simulink model "DYC_DLCtight_Fuzzy_and_NN_prediction"  (Simulink 8.9)
settings: Solver=VariableStepAuto  StartTime=0  StopTime=8  FixedStep=0.001  RelTol=1e-3  AbsTol=1e-6
libraries: neural x138, fuzblock x6, dspfdesign x6, Solver_SF x1, simulink x1
(part 1 of 4)
settings Model: Creator=ywata  LastModifiedBy=Huang Guoming  ExtModeTrigMode=oneshot  ExtModeArmWhenConnect=off
settings Model: LogicAnalyzerGraphicalSettings=|
  | {
  |   "cursors" : {
  |     "activeCursor" : 1,
  |     "lockedCursors" : [
  | 
  |     ],
  |     "startingCursor" : 0,
  |     "times" : [
  |       1.76,
  |       0.487,
  |       1.4983333333333333
  |     ]
  |   },
  |   "global" : {
  |   },
  |   "panels" : [
  |     {
  |       "height" : 100,
  |       "startingTrace" : 0,
  |       "traces" : [
  | 
  |       ],
  |       "yOffset" : 0
  |     }
  |   ],
  |   "timeAxis" : {
  |     "pixelsPerSecond" : 300
  |   }
  | }
settings DataIOCC: LimitDataPoints=off  SignalLoggingName=sigsOut
settings OptimizationCC: BooleanDataType=off
settings DebuggingCC: SaveWithParameterizedLinksMsg=none  SignalResolutionControl=TryResolveAllWithWarning  MultiTaskDSMMsg=warning  MultiTaskCondExecSysMsg=none
settings HardwareCC: TargetBitPerPointer=64  TargetBitPerSizeT=64  TargetBitPerPtrDiffT=64  TargetLongLongMode=on  TargetIntDivRoundTo=Zero  TargetEndianess=LittleEndian  TargetWordSize=64  TargetHWDeviceType=MATLAB Host  ProdEqTarget=off
settings RTWCC: TemplateMakefile=grt_vc.tmf
settings GRTTargetCC: GeneratePreprocessorConditionals=Use local settings

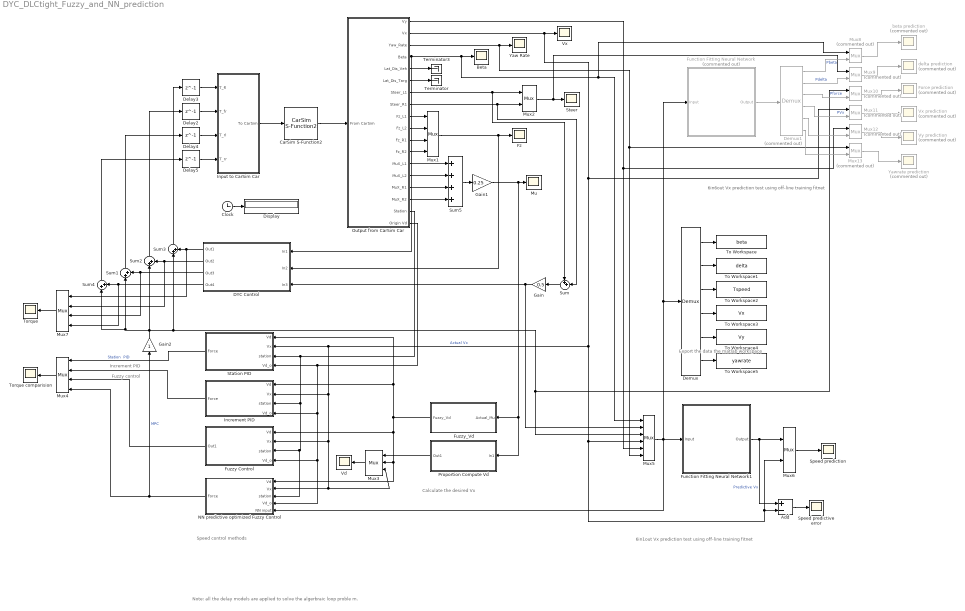
== system DYC_DLCtight_Fuzzy_and_NN_prediction ==
  note: Fuzzy control
  note: Increment PID
  note: Calculate the desired Vx
  note: Speed control methods
  note: Export the data the matlab workspace
  note: Note: all the delay models are applied to solve the algerbraic loop proble m.
  note: 6in1out Vx prediction test using off-line training fitnet
  note: 6in6out Vx prediction test using off-line training fitnet
  " Force prediction" : Scope  Commented=on
  " Fuzzy Control" : Subsystem
      mask Display: image('fuzzy.jpg');
  " Vx prediction" : Scope  Commented=on
  " Vy prediction" : Scope  Commented=on
  " Yawrate prediction" : Scope  Commented=on
  " beta prediction" : Scope  Commented=on
  " delta prediction" : Scope  Commented=on
  Add : Sum  Inputs=+-
  Beta : Scope
  CarSim S-Function2 : Solver_SF/CarSim S-Function2  Priority=1  VehicleCode=i_i  SIMFILE=simfile.sim
      settings: AttributesFormatString=Vehicle Code: %<VehicleCode>
  Clock : Clock
  DYC Control : Subsystem
  Delay{2..5} (4 alike) : Delay  DelayLength=1  InitialCondition=0  SampleTime=0.001
  Demux : Demux  Outputs=6
  Demux1 : Demux  Commented=on  Outputs=6
  Display : Display
      settings: Format=bank  Decimation=100
  Function Fitting Neural Network : Subsystem  Commented=on
      mask help: Function Fitting Neural Network
      mask Display: e = 0.06;c1 = [120 150 230]/255;c2 = ([120 150 230]+0)/383;c3 = ([120 150 230]+128)/383;patch([0 1 1 0],[0 0 1 1],c1);patch([0 1 1 1-e 1-e 0+e],[0 0 1 1-e 0+e 0+e],c2);patch([0 0 1 1-e 0+e 0+e],[0 1 1 1-e 1-e 0+e],c3);plot([0 1 1 0 0],[0 0 1 1 0]);fprintf('NNET');port_label('input',1,' Input');port_label('output',1,'Output ');
  Function Fitting Neural Network1 : Subsystem
      mask help: Function Fitting Neural Network
      mask Display: e = 0.06;c1 = [120 150 230]/255;c2 = ([120 150 230]+0)/383;c3 = ([120 150 230]+128)/383;patch([0 1 1 0],[0 0 1 1],c1);patch([0 1 1 1-e 1-e 0+e],[0 0 1 1-e 0+e 0+e],c2);patch([0 0 1 1-e 0+e 0+e],[0 1 1 1-e 1-e 0+e],c3);plot([0 1 1 0 0],[0 0 1 1 0]);fprintf('NNET');port_label('input',1,' Input');port_label('output',1,'Output ');
  Fuzzy_Vd : MATLAB Function  TreatAsAtomicUnit=on
  Fz : Scope
  Gain : Gain  Gain=0.5
  Gain1 : Gain  Gain=0.25
  Gain2 : Gain
  "Increment PID " : Subsystem
  Input to CarSim Car : Subsystem
  Mu : Scope
  Mux1 : Mux
  Mux{8..13} (6 alike) : Mux  Commented=on  Inputs=2
  Mux2 : Mux  Inputs=2
  Mux3 : Mux  Inputs=3
  Mux4 : Mux
  Mux5 : Mux  Inputs=6
  Mux6 : Mux  Inputs=2
  Mux7 : Mux
  NN predictive optimized Fuzzy Control : Subsystem
  Output from CarSim Car : Subsystem
  Proportion Compute Vd : Subsystem
  Speed prediction : Scope
  Speed predictive error : Scope
  Station PID : Subsystem
  Steer : Scope
  Sum : Sum  Inputs=++|
  Sum{1..4} (4 alike) : Sum  Inputs=|++
  Sum5 : Sum  Inputs=++++
  Terminator : Terminator
  Terminator3 : Terminator
  To Workspace : ToWorkspace  VariableName=beta  SampleTime=-1
      settings: Save2DSignal=2-D array (concatenate along first dimension)
  To Workspace1 : ToWorkspace  VariableName=delta  SampleTime=-1
      settings: Save2DSignal=2-D array (concatenate along first dimension)
  To Workspace2 : ToWorkspace  VariableName=Tspeed  SampleTime=-1
      settings: Save2DSignal=2-D array (concatenate along first dimension)
  To Workspace3 : ToWorkspace  VariableName=Vx  SampleTime=-1
      settings: Save2DSignal=2-D array (concatenate along first dimension)
  To Workspace4 : ToWorkspace  VariableName=Vy  SampleTime=-1
      settings: Save2DSignal=2-D array (concatenate along first dimension)
  To Workspace5 : ToWorkspace  VariableName=yawrate  SampleTime=-1
      settings: Save2DSignal=2-D array (concatenate along first dimension)
  Torque : Scope
  Torque comparision : Scope
  Vd : Scope
  Vx : Scope
  Yaw Rate : Scope
  wires:
  Clock/1 -> Display/1
  Mux2/1 -> Mux9/1, Steer/1
  Mux7/1 -> Torque/1
  Output from CarSim Car/3(Yaw_Rate) -> Mux5/6, Mux13/1, Yaw Rate/1
  Output from CarSim Car/6(Lat_Dis_Targ) -> Terminator/1
  Output from CarSim Car/5(Lat_Dis_Veh) -> Terminator3/1
  Output from CarSim Car/1(Vy) -> Mux5/5, Mux12/1
  Output from CarSim Car/4(Beta) -> Mux8/1, Mux5/1, Beta/1, DYC Control/1(In1)
  Output from CarSim Car/7(Steer_L1) -> Sum/1, Mux2/1
  Output from CarSim Car/8(Steer_R1) -> Sum/2, Mux2/2
  Output from CarSim Car/2(Vx) -> Mux11/1, Mux3/3, NN predictive optimized Fuzzy Control/2(Vx), " Fuzzy Control"/2(Vx), "Increment PID "/2(Vx), Station PID/2(Vx), Mux5/4, Mux6/2, Add/2, Vx/1  "Actual Vx"
  Sum/1 -> Gain/1
  Sum3/1 -> Delay3/1
  Sum2/1 -> Delay2/1
  Sum4/1 -> Delay5/1
  Output from CarSim Car/13(MuX_L1) -> Sum5/1
  Output from CarSim Car/14(MuX_L2) -> Sum5/2
  Output from CarSim Car/15(MuX_R1) -> Sum5/3
  Output from CarSim Car/16(MuX_R2) -> Sum5/4
  Sum5/1 -> Gain1/1
  Gain1/1 -> Mu/1, Fuzzy_Vd/1(Actual_Mu), Proportion Compute Vd/1(In1)
  CarSim S-Function2/1 -> Output from CarSim Car/1(From CarSim)
  Input to CarSim Car/1(To CarSim) -> CarSim S-Function2/1
  Output from CarSim Car/9(Fz_L1) -> Mux1/1
  Output from CarSim Car/10(Fz_L2) -> Mux1/2
  Output from CarSim Car/11(Fz_R1) -> Mux1/3
  Output from CarSim Car/12(Fz_R2) -> Mux1/4
  Mux1/1 -> DYC Control/2(In2), Fz/1
  Mux3/1 -> Vd/1
  Proportion Compute Vd/1(Out1) -> Mux3/1
  Mux4/1 -> Torque comparision/1
  Delay3/1 -> Input to CarSim Car/1(T_fl)
  Delay2/1 -> Input to CarSim Car/2(T_fr)
  Delay4/1 -> Input to CarSim Car/3(T_rl)
  Delay5/1 -> Input to CarSim Car/4(T_rr)
  DYC Control/2(Out2) -> Sum2/2, Mux7/2
  DYC Control/4(Out4) -> Sum4/2, Mux7/4
  DYC Control/1(Out1) -> Sum3/2, Mux7/1
  DYC Control/3(Out3) -> Sum1/2, Mux7/3
  Gain/1 -> Mux5/2, DYC Control/3(In3)
  Station PID/1(Force) -> Mux4/1  "Station  PID"
  Sum1/1 -> Delay4/1
  Function Fitting Neural Network1/1(Output) -> Add/1, Mux6/1  "Predictive Vx"
  Mux6/1 -> Speed prediction/1
  " Fuzzy Control"/1(Out1) -> Mux4/3
  Demux/5 -> To Workspace4/1
  Demux/4 -> To Workspace3/1
  Demux/3 -> To Workspace2/1
  Demux/2 -> To Workspace1/1
  Demux/1 -> To Workspace/1
  Demux/6 -> To Workspace5/1
  Mux5/1 -> Function Fitting Neural Network/1(Input), Demux/1, NN predictive optimized Fuzzy Control/5(NN input), Function Fitting Neural Network1/1(Input)
  Gain2/1 -> Sum4/1, Sum1/1, Sum2/1, Mux10/1, Mux5/3, Sum3/1
  "Increment PID "/1(Force) -> Mux4/2
  Add/1 -> Speed predictive error/1
  Fuzzy_Vd/1(Fuzzy_Vd) -> Station PID/1(Vd), "Increment PID "/1(Vd), NN predictive optimized Fuzzy Control/1(Vd), Mux3/2, " Fuzzy Control"/1(Vd)
  Output from CarSim Car/18(Origin Vd) -> NN predictive optimized Fuzzy Control/4(Vd_o), " Fuzzy Control"/4(Vd_o), "Increment PID "/4(Vd_o), Station PID/4(Vd_o)
  Output from CarSim Car/17(Station) -> NN predictive optimized Fuzzy Control/3(station), " Fuzzy Control"/3(station), "Increment PID "/3(station), Station PID/3(station)
  NN predictive optimized Fuzzy Control/1(Force) -> Gain2/1, Mux4/4  "MPC"
  Function Fitting Neural Network/1(Output) -> Demux1/1
  Mux8/1 -> " beta prediction"/1
  Demux1/1 -> Mux8/2  "Pbeta"
  Demux1/2 -> Mux9/2  "Pdelta"
  Mux9/1 -> " delta prediction"/1
  Demux1/3 -> Mux10/2  "Pforce"
  Mux10/1 -> " Force prediction"/1
  Demux1/4 -> Mux11/2  "PVx"
  Mux11/1 -> " Vx prediction"/1
  Demux1/5 -> Mux12/2
  Mux12/1 -> " Vy prediction"/1
  Demux1/6 -> Mux13/2
  Mux13/1 -> " Yawrate prediction"/1

== system DYC_DLCtight_Fuzzy_and_NN_prediction/ Fuzzy Control ==
  Vd : Inport
  Vx : Inport  Port=2
  station : Inport  Port=3
  Vd_o : Inport  Port=4
  Fuzzy control : Subsystem
  Select Vd : MATLAB Function  TreatAsAtomicUnit=on
  Out1 : Outport
  wires:
  Fuzzy control/1(Out1) -> Out1/1
  Select Vd/1(Ve) -> Fuzzy control/1(In1)
  Vd/1 -> Select Vd/1(Vd)
  Vx/1 -> Select Vd/2(Vx)
  station/1 -> Select Vd/3(station)
  Vd_o/1 -> Select Vd/4(Vd_o)

== system DYC_DLCtight_Fuzzy_and_NN_prediction/DYC Control ==
  In1 : Inport
  In2 : Inport  Port=2
  In3 : Inport  Port=3
  DYC  control method : MATLAB Function  TreatAsAtomicUnit=on
  Demux : Demux
  Out1 : Outport
  Out2 : Outport  Port=2
  Out3 : Outport  Port=3
  Out4 : Outport  Port=4
  wires:
  In3/1 -> DYC  control method/1(delta)
  DYC  control method/1(T1) -> Out1/1
  Demux/2 -> DYC  control method/4(Fz_fr)
  DYC  control method/4(T4) -> Out4/1
  Demux/1 -> DYC  control method/3(Fz_fl)
  Demux/4 -> DYC  control method/6(Fz_rr)
  DYC  control method/3(T3) -> Out3/1
  DYC  control method/2(T2) -> Out2/1
  Demux/3 -> DYC  control method/5(Fz_rl)
  In2/1 -> Demux/1
  In1/1 -> DYC  control method/2(beta)

== system DYC_DLCtight_Fuzzy_and_NN_prediction/Function Fitting Neural Network ==
  Input : Inport  PortDimensions=6
      mask Display: e = 0.06;c1 = [120 230 180]/255;c2 = ([120 230 180]+0)/(256+128);c3 = ([120 230 180]+128)/(256+128);patch([0 1 1 0],[0 0 1 1],c1);patch([0 1 1 1-e 1-e 0+e],[0 0 1 1-e 0+e 0+e],c2);patch([0 0 1 1-e 0+e 0+e],[0 1 1 1-e 1-e 0+e],c3);plot([0 1 1 0 0],[0 0 1 1 0]);
  Layer 1 : Subsystem
      mask Display: e = 0.06;c1 = [120 150 230]/255;c2 = ([120 150 230]+0)/383;c3 = ([120 150 230]+128)/383;patch([0 1 1 0],[0 0 1 1],c1);patch([0 1 1 1-e 1-e 0+e],[0 0 1 1-e 0+e 0+e],c2);patch([0 0 1 1-e 0+e 0+e],[0 1 1 1-e 1-e 0+e],c3);plot([0 1 1 0 0],[0 0 1 1 0]);
  Layer 2 : Subsystem
      mask Display: e = 0.06;c1 = [120 150 230]/255;c2 = ([120 150 230]+0)/383;c3 = ([120 150 230]+128)/383;patch([0 1 1 0],[0 0 1 1],c1);patch([0 1 1 1-e 1-e 0+e],[0 0 1 1-e 0+e 0+e],c2);patch([0 0 1 1-e 0+e 0+e],[0 1 1 1-e 1-e 0+e],c3);plot([0 1 1 0 0],[0 0 1 1 0]);
  Process Input 1 : Subsystem
      mask Display: e = 0.06;c1 = [120 150 230]/255;c2 = ([120 150 230]+0)/383;c3 = ([120 150 230]+128)/383;patch([0 1 1 0],[0 0 1 1],c1);patch([0 1 1 1-e 1-e 0+e],[0 0 1 1-e 0+e 0+e],c2);patch([0 0 1 1-e 0+e 0+e],[0 1 1 1-e 1-e 0+e],c3);plot([0 1 1 0 0],[0 0 1 1 0]);
  Process Output 1 : Subsystem
      mask Display: e = 0.06;c1 = [120 150 230]/255;c2 = ([120 150 230]+0)/383;c3 = ([120 150 230]+128)/383;patch([0 1 1 0],[0 0 1 1],c1);patch([0 1 1 1-e 1-e 0+e],[0 0 1 1-e 0+e 0+e],c2);patch([0 0 1 1-e 0+e 0+e],[0 1 1 1-e 1-e 0+e],c3);plot([0 1 1 0 0],[0 0 1 1 0]);
  Output : Outport  InitialOutput=[0;0;0;0;0;0]
      mask Display: e = 0.06;c1 = [120 230 180]/255;c2 = ([120 230 180]+0)/(256+128);c3 = ([120 230 180]+128)/(256+128);patch([0 1 1 0],[0 0 1 1],c1);patch([0 1 1 1-e 1-e 0+e],[0 0 1 1-e 0+e 0+e],c2);patch([0 0 1 1-e 0+e 0+e],[0 1 1 1-e 1-e 0+e],c3);plot([0 1 1 0 0],[0 0 1 1 0]);
  wires:
  Input/1 -> Process Input 1/1(x)
  Process Output 1/1(y) -> Output/1
  Process Input 1/1(p) -> Layer 1/1("p{1}")
  Layer 1/1("a{1}") -> [feedback1]
  [feedback1] -> Layer 2/1("a{1} ")
  Layer 2/1("a{2}") -> Process Output 1/1(a)

== system DYC_DLCtight_Fuzzy_and_NN_prediction/Function Fitting Neural Network1 ==
  Input : Inport  PortDimensions=6
      mask Display: e = 0.06;c1 = [120 230 180]/255;c2 = ([120 230 180]+0)/(256+128);c3 = ([120 230 180]+128)/(256+128);patch([0 1 1 0],[0 0 1 1],c1);patch([0 1 1 1-e 1-e 0+e],[0 0 1 1-e 0+e 0+e],c2);patch([0 0 1 1-e 0+e 0+e],[0 1 1 1-e 1-e 0+e],c3);plot([0 1 1 0 0],[0 0 1 1 0]);
  Layer 1 : Subsystem
      mask Display: e = 0.06;c1 = [120 150 230]/255;c2 = ([120 150 230]+0)/383;c3 = ([120 150 230]+128)/383;patch([0 1 1 0],[0 0 1 1],c1);patch([0 1 1 1-e 1-e 0+e],[0 0 1 1-e 0+e 0+e],c2);patch([0 0 1 1-e 0+e 0+e],[0 1 1 1-e 1-e 0+e],c3);plot([0 1 1 0 0],[0 0 1 1 0]);
  Layer 2 : Subsystem
      mask Display: e = 0.06;c1 = [120 150 230]/255;c2 = ([120 150 230]+0)/383;c3 = ([120 150 230]+128)/383;patch([0 1 1 0],[0 0 1 1],c1);patch([0 1 1 1-e 1-e 0+e],[0 0 1 1-e 0+e 0+e],c2);patch([0 0 1 1-e 0+e 0+e],[0 1 1 1-e 1-e 0+e],c3);plot([0 1 1 0 0],[0 0 1 1 0]);
  Process Input 1 : Subsystem
      mask Display: e = 0.06;c1 = [120 150 230]/255;c2 = ([120 150 230]+0)/383;c3 = ([120 150 230]+128)/383;patch([0 1 1 0],[0 0 1 1],c1);patch([0 1 1 1-e 1-e 0+e],[0 0 1 1-e 0+e 0+e],c2);patch([0 0 1 1-e 0+e 0+e],[0 1 1 1-e 1-e 0+e],c3);plot([0 1 1 0 0],[0 0 1 1 0]);
  Process Output 1 : Subsystem
      mask Display: e = 0.06;c1 = [120 150 230]/255;c2 = ([120 150 230]+0)/383;c3 = ([120 150 230]+128)/383;patch([0 1 1 0],[0 0 1 1],c1);patch([0 1 1 1-e 1-e 0+e],[0 0 1 1-e 0+e 0+e],c2);patch([0 0 1 1-e 0+e 0+e],[0 1 1 1-e 1-e 0+e],c3);plot([0 1 1 0 0],[0 0 1 1 0]);
  Output : Outport  InitialOutput=0
      mask Display: e = 0.06;c1 = [120 230 180]/255;c2 = ([120 230 180]+0)/(256+128);c3 = ([120 230 180]+128)/(256+128);patch([0 1 1 0],[0 0 1 1],c1);patch([0 1 1 1-e 1-e 0+e],[0 0 1 1-e 0+e 0+e],c2);patch([0 0 1 1-e 0+e 0+e],[0 1 1 1-e 1-e 0+e],c3);plot([0 1 1 0 0],[0 0 1 1 0]);
  wires:
  Input/1 -> Process Input 1/1(x)
  Process Output 1/1(y) -> Output/1
  Process Input 1/1(p) -> Layer 1/1("p{1}")
  Layer 1/1("a{1}") -> [feedback1]
  [feedback1] -> Layer 2/1("a{1} ")
  Layer 2/1("a{2}") -> Process Output 1/1(a)

== system DYC_DLCtight_Fuzzy_and_NN_prediction/Increment PID  ==
  Vd : Inport
  Vx : Inport  Port=2
  station : Inport  Port=3
  Vd_o : Inport  Port=4
  "Increment PID " : Subsystem
  Select Vd : MATLAB Function  TreatAsAtomicUnit=on
  Force : Outport
  wires:
  "Increment PID "/1(Out1) -> Force/1
  Select Vd/1(Ve) -> "Increment PID "/1(In1)
  Vd/1 -> Select Vd/1(Vd)
  Vx/1 -> Select Vd/2(Vx)
  station/1 -> Select Vd/3(station)
  Vd_o/1 -> Select Vd/4(Vd_o)

== system DYC_DLCtight_Fuzzy_and_NN_prediction/Input to CarSim Car ==
  T_fl : Inport
  T_fr : Inport  Port=2
  T_rl : Inport  Port=3
  T_rr : Inport  Port=4
  Mux : Mux
  To CarSim : Outport
  wires:
  T_rr/1 -> Mux/4
  T_rl/1 -> Mux/3
  T_fr/1 -> Mux/2
  T_fl/1 -> Mux/1
  Mux/1 -> To CarSim/1

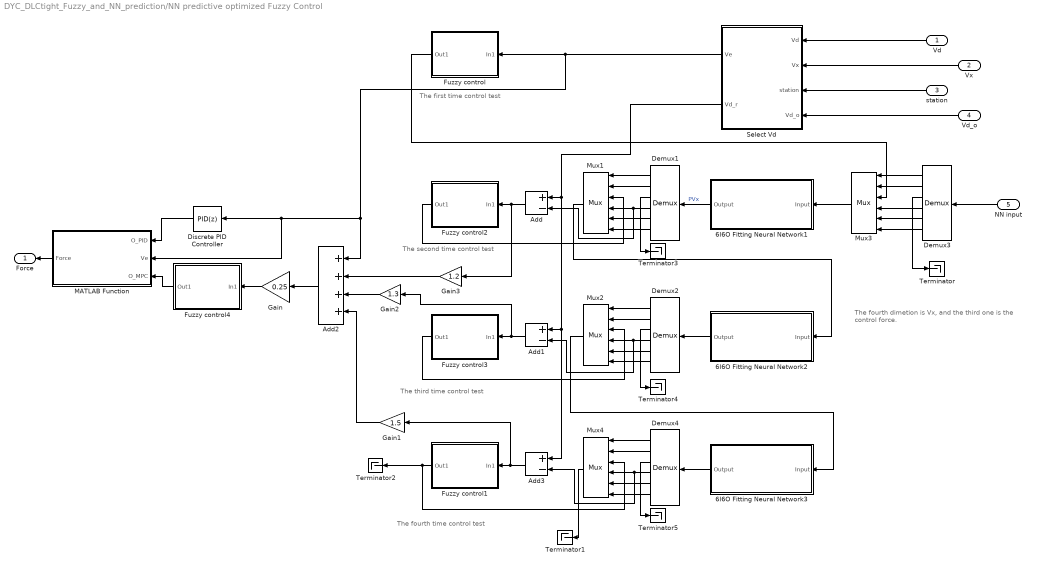
== system DYC_DLCtight_Fuzzy_and_NN_prediction/NN predictive optimized Fuzzy Control ==
  note: The first time control test
  note: The fourth dimetion is Vx,
      | and the third one is the control force.
  note: The second time control test
  note: The third time control test
  note: The fourth time control test
  Vd : Inport
  Vx : Inport  Port=2
  station : Inport  Port=3
  Vd_o : Inport  Port=4
  NN input : Inport  Port=5
  6I6O Fitting Neural Network1 : Subsystem
      mask help: Function Fitting Neural Network
      mask Display: e = 0.06;c1 = [120 150 230]/255;c2 = ([120 150 230]+0)/383;c3 = ([120 150 230]+128)/383;patch([0 1 1 0],[0 0 1 1],c1);patch([0 1 1 1-e 1-e 0+e],[0 0 1 1-e 0+e 0+e],c2);patch([0 0 1 1-e 0+e 0+e],[0 1 1 1-e 1-e 0+e],c3);plot([0 1 1 0 0],[0 0 1 1 0]);fprintf('NNET');port_label('input',1,' Input');port_label('output',1,'Output ');
  6I6O Fitting Neural Network2 : Subsystem
      mask help: Function Fitting Neural Network
      mask Display: e = 0.06;c1 = [120 150 230]/255;c2 = ([120 150 230]+0)/383;c3 = ([120 150 230]+128)/383;patch([0 1 1 0],[0 0 1 1],c1);patch([0 1 1 1-e 1-e 0+e],[0 0 1 1-e 0+e 0+e],c2);patch([0 0 1 1-e 0+e 0+e],[0 1 1 1-e 1-e 0+e],c3);plot([0 1 1 0 0],[0 0 1 1 0]);fprintf('NNET');port_label('input',1,' Input');port_label('output',1,'Output ');
  6I6O Fitting Neural Network3 : Subsystem
      mask help: Function Fitting Neural Network
      mask Display: e = 0.06;c1 = [120 150 230]/255;c2 = ([120 150 230]+0)/383;c3 = ([120 150 230]+128)/383;patch([0 1 1 0],[0 0 1 1],c1);patch([0 1 1 1-e 1-e 0+e],[0 0 1 1-e 0+e 0+e],c2);patch([0 0 1 1-e 0+e 0+e],[0 1 1 1-e 1-e 0+e],c3);plot([0 1 1 0 0],[0 0 1 1 0]);fprintf('NNET');port_label('input',1,' Input');port_label('output',1,'Output ');
  Add : Sum  Inputs=+-
  Add1 : Sum  Inputs=+-
  Add2 : Sum  Inputs=++++
  Add3 : Sum  Inputs=+-
  Demux{1..4} (4 alike) : Demux  Outputs=6
  Discrete PID Controller : simulink/Continuous/PID Controller  Controller=PID  TimeDomain=Discrete-time  SampleTime=-1  IntegratorMethod=Forward Euler  FilterMethod=Forward Euler  Form=Parallel  UseFilter=on  ControllerParametersSource=internal  P=500  I=0  D=200  N=100  InitialConditionSource=internal  InitialConditionForIntegrator=0  InitialConditionForFilter=0  ExternalReset=none  LimitOutput=off  UpperSaturationLimit=inf  LowerSaturationLimit=-inf  LinearizeAsGain=off  AntiWindupMode=none  Kb=1  TrackingMode=off  Kt=1  PParamMin=[]  PParamMax=[]  IParamMin=[]  IParamMax=[]  DParamMin=[]  DParamMax=[]  NParamMin=[]  NParamMax=[]  KbParamMin=[]  KbParamMax=[]  KtParamMin=[]  KtParamMax=[]  POutMin=[]  POutMax=[]  IOutMin=[]  IOutMax=[]  DOutMin=[]  DOutMax=[]  NOutMin=[]  NOutMax=[]  KbOutMin=[]  KbOutMax=[]  KtOutMin=[]  KtOutMax=[]  IntegratorOutMin=[]  IntegratorOutMax=[]  FilterOutMin=[]  FilterOutMax=[]  SumOutMin=[]  SumOutMax=[]  SumI1OutMin=[]  SumI1OutMax=[]  SumI2OutMin=[]  SumI2OutMax=[]  SumI3OutMin=[]  SumI3OutMax=[]  SumDOutMin=[]  SumDOutMax=[]  SaturationOutMin=[]  SaturationOutMax=[]  IntegratorContinuousStateAttributes=''  IntegratorStateMustResolveToSignalObject=off  IntegratorRTWStateStorageClass=Auto  FilterContinuousStateAttributes=''  FilterStateMustResolveToSignalObject=off  FilterRTWStateStorageClass=Auto  DifferentiatorICPrevScaledInput=0  DifferentiatorOutMin=[]  DifferentiatorOutMax=[]  InitialConditionSetting=State (most efficient)
  Fuzzy control : Subsystem
  Fuzzy control1 : Subsystem
  Fuzzy control2 : Subsystem
  Fuzzy control3 : Subsystem
  Fuzzy control4 : Subsystem
  Gain : Gain  Gain=0.25
  Gain1 : Gain  Gain=1.5
  Gain2 : Gain  Gain=1.3
  Gain3 : Gain  Gain=1.2
  MATLAB Function : MATLAB Function  TreatAsAtomicUnit=on
  Mux{1..4} (4 alike) : Mux  Inputs=6
  Select Vd : MATLAB Function  TreatAsAtomicUnit=on
  Terminator{,1..5} (6 alike) : Terminator
  Force : Outport
  wires:
  Vd_o/1 -> Select Vd/4(Vd_o)
  station/1 -> Select Vd/3(station)
  Vx/1 -> Select Vd/2(Vx)
  Vd/1 -> Select Vd/1(Vd)
  6I6O Fitting Neural Network1/1(Output) -> Demux1/1  "PVx"
  Mux1/1 -> 6I6O Fitting Neural Network2/1(Input)
  Demux1/6 -> Mux1/6
  Demux1/5 -> Mux1/5
  Demux1/2 -> Mux1/2
  Demux1/1 -> Mux1/1
  Select Vd/1(Ve) -> MATLAB Function/2(Ve), Discrete PID Controller/1, Add2/1, Fuzzy control/1(In1)
  Demux2/1 -> Mux2/1
  Demux2/2 -> Mux2/2
  Demux2/5 -> Mux2/5
  Demux2/6 -> Mux2/6
  6I6O Fitting Neural Network2/1(Output) -> Demux2/1
  NN input/1 -> Demux3/1
  Mux3/1 -> 6I6O Fitting Neural Network1/1(Input)
  Demux3/5 -> Mux3/5
  Demux3/6 -> Mux3/6
  Demux3/2 -> Mux3/2
  Demux3/1 -> Mux3/1
  Add/1 -> Gain3/1, Fuzzy control2/1(In1)
  Add1/1 -> Gain2/1, Fuzzy control3/1(In1)
  6I6O Fitting Neural Network3/1(Output) -> Demux4/1
  Demux4/6 -> Mux4/6
  Demux4/5 -> Mux4/5
  Demux4/2 -> Mux4/2
  Demux4/1 -> Mux4/1
  Mux2/1 -> 6I6O Fitting Neural Network3/1(Input)
  Select Vd/2(Vd_r) -> Add1/1, Add3/1, Add/1
  Add3/1 -> Gain1/1, Fuzzy control1/1(In1)
  Mux4/1 -> Terminator1/1
  Add2/1 -> Gain/1
  Gain/1 -> Fuzzy control4/1(In1)
  Demux2/4 -> Add1/2, Mux2/4
  Fuzzy control3/1(Out1) -> Mux2/3
  Demux4/4 -> Add3/2, Mux4/4
  Fuzzy control/1(Out1) -> Mux3/3
  Demux3/4 -> Mux3/4
  Demux3/3 -> Terminator/1
  Fuzzy control2/1(Out1) -> Mux1/3
  Fuzzy control1/1(Out1) -> Mux4/3, Terminator2/1
  Demux1/4 -> Mux1/4, Add/2
  Demux1/3 -> Terminator3/1
  Demux2/3 -> Terminator4/1
  Demux4/3 -> Terminator5/1
  Gain1/1 -> Add2/4
  Gain2/1 -> Add2/3
  Gain3/1 -> Add2/2
  Fuzzy control4/1(Out1) -> MATLAB Function/3(O_MPC)
  MATLAB Function/1(Force) -> Force/1
  Discrete PID Controller/1 -> MATLAB Function/1(O_PID)

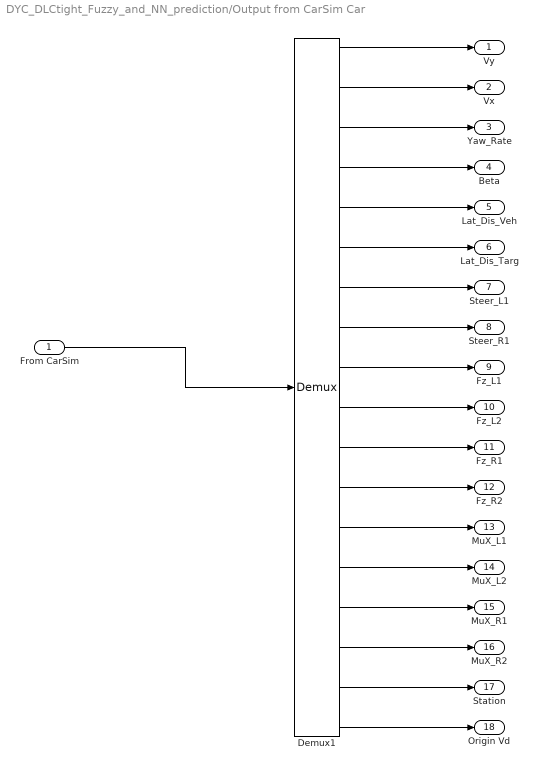
== system DYC_DLCtight_Fuzzy_and_NN_prediction/Output from CarSim Car ==
  From CarSim : Inport
  Demux1 : Demux  Outputs=18
  Vy : Outport
  Vx : Outport  Port=2
  Yaw_Rate : Outport  Port=3
  Beta : Outport  Port=4
  Lat_Dis_Veh : Outport  Port=5
  Lat_Dis_Targ : Outport  Port=6
  Steer_L1 : Outport  Port=7
  Steer_R1 : Outport  Port=8
  Fz_L1 : Outport  Port=9
  Fz_L2 : Outport  Port=10
  Fz_R1 : Outport  Port=11
  Fz_R2 : Outport  Port=12
  MuX_L1 : Outport  Port=13
  MuX_L2 : Outport  Port=14
  MuX_R1 : Outport  Port=15
  MuX_R2 : Outport  Port=16
  Station : Outport  Port=17
  Origin Vd : Outport  Port=18
  wires:
  From CarSim/1 -> Demux1/1
  Demux1/2 -> Vx/1
  Demux1/3 -> Yaw_Rate/1
  Demux1/1 -> Vy/1
  Demux1/8 -> Steer_R1/1
  Demux1/4 -> Beta/1
  Demux1/5 -> Lat_Dis_Veh/1
  Demux1/6 -> Lat_Dis_Targ/1
  Demux1/7 -> Steer_L1/1
  Demux1/9 -> Fz_L1/1
  Demux1/10 -> Fz_L2/1
  Demux1/11 -> Fz_R1/1
  Demux1/12 -> Fz_R2/1
  Demux1/13 -> MuX_L1/1
  Demux1/14 -> MuX_L2/1
  Demux1/15 -> MuX_R1/1
  Demux1/16 -> MuX_R2/1
  Demux1/17 -> Station/1
  Demux1/18 -> Origin Vd/1

== system DYC_DLCtight_Fuzzy_and_NN_prediction/Proportion Compute Vd ==
  In1 : Inport
  Constant : Constant  Value=0.45
  Constant1 : Constant  Value=30
  Gain : Gain  Gain=50
  Sum : Sum  Inputs=|+-
  Sum1 : Sum
  Out1 : Outport
  wires:
  In1/1 -> Sum/1
  Constant/1 -> Sum/2
  Sum/1 -> Gain/1
  Gain/1 -> Sum1/1
  Sum1/1 -> Out1/1
  Constant1/1 -> Sum1/2

== system DYC_DLCtight_Fuzzy_and_NN_prediction/Station PID ==
  Vd : Inport
  Vx : Inport  Port=2
  station : Inport  Port=3
  Vd_o : Inport  Port=4
  " PID speed control method" : MATLAB Function  TreatAsAtomicUnit=on
  Force : Outport
  wires:
  " PID speed control method"/1(BrakeTorque) -> Force/1
  Vd/1 -> " PID speed control method"/1(Vd)
  Vx/1 -> " PID speed control method"/2(Vx)
  Vd_o/1 -> " PID speed control method"/4(Vd_o)
  station/1 -> " PID speed control method"/3(station)

== system DYC_DLCtight_Fuzzy_and_NN_prediction/ Fuzzy Control/Fuzzy control ==
  In1 : Inport
  Fuzzy Logic  Controller : fuzblock/Fuzzy Logic  Controller  fis='FuzzyInferenceSystem.fis'
  Gain3 : Gain  Gain=120
  Signal pre-process : Subsystem
  Out1 : Outport
  wires:
  Gain3/1 -> Out1/1
  Signal pre-process/1(Out1) -> Fuzzy Logic  Controller/1
  In1/1 -> Signal pre-process/1(In1)
  Fuzzy Logic  Controller/1 -> Gain3/1

== system DYC_DLCtight_Fuzzy_and_NN_prediction/Function Fitting Neural Network/Layer 1 ==
  "p{1}" : Inport  PortDimensions=6
      mask Display: e = 0.06;c1 = [120 230 180]/255;c2 = ([120 230 180]+0)/(256+128);c3 = ([120 230 180]+128)/(256+128);patch([0 1 1 0],[0 0 1 1],c1);patch([0 1 1 1-e 1-e 0+e],[0 0 1 1-e 0+e 0+e],c2);patch([0 0 1 1-e 0+e 0+e],[0 1 1 1-e 1-e 0+e],c3);plot([0 1 1 0 0],[0 0 1 1 0]);
  Delays 1 : Subsystem
      mask Display: e = 0.06;c1 = [120 150 230]/255;c2 = ([120 150 230]+0)/383;c3 = ([120 150 230]+128)/383;patch([0 1 1 0],[0 0 1 1],c1);patch([0 1 1 1-e 1-e 0+e],[0 0 1 1-e 0+e 0+e],c2);patch([0 0 1 1-e 0+e 0+e],[0 1 1 1-e 1-e 0+e],c3);plot([0 1 1 0 0],[0 0 1 1 0]);disp('0');
  "IW{1,1}" : Subsystem
      mask Display: e = 0.06;c1 = [120 150 230]/255;c2 = ([120 150 230]+0)/383;c3 = ([120 150 230]+128)/383;patch([0 1 1 0],[0 0 1 1],c1);patch([0 1 1 1-e 1-e 0+e],[0 0 1 1-e 0+e 0+e],c2);patch([0 0 1 1-e 0+e 0+e],[0 1 1 1-e 1-e 0+e],c3);plot([0 1 1 0 0],[0 0 1 1 0]);disp('W');
  "b{1}" : Constant  Value=[0.6879967300188552;0.77057293695217965;-1.6023960110469773;0.76890651286062883;0.69835683605814192;1.3234515610986295;-0.44999046297264095;0.55787593212697362;-0.26419195749866425;-0.019958997340300579;-0.11355214173111271;0.56452123367098961;-0.031853380480054747;-0.54673650323643108;0.63578729872957629;1.7653302338217376;0.91957766891446979;-0.75733275821037604;-0.70013712007031903;2.9214372511806581]
      mask Display: e = 0.06;c1 = [120 150 230]/255;c2 = ([120 150 230]+0)/383;c3 = ([120 150 230]+128)/383;patch([0 1 1 0],[0 0 1 1],c1);patch([0 1 1 1-e 1-e 0+e],[0 0 1 1-e 0+e 0+e],c2);patch([0 0 1 1-e 0+e 0+e],[0 1 1 1-e 1-e 0+e],c3);plot([0 1 1 0 0],[0 0 1 1 0]);disp('b');
  netsum : Sum  Inputs=2  SaturateOnIntegerOverflow=on  InputSameDT=on  OutDataTypeStr=Inherit: Same as first input
      mask Display: e = 0.06;c1 = [120 150 230]/255;c2 = ([120 150 230]+0)/383;c3 = ([120 150 230]+128)/383;patch([0 1 1 0],[0 0 1 1],c1);patch([0 1 1 1-e 1-e 0+e],[0 0 1 1-e 0+e 0+e],c2);patch([0 0 1 1-e 0+e 0+e],[0 1 1 1-e 1-e 0+e],c3);plot([0 1 1 0 0],[0 0 1 1 0]);disp('+');
  tansig : neural/Transfer Functions/tansig
  "a{1}" : Outport  InitialOutput=[0;0;0;0;0;0;0;0;0;0;0;0;0;0;0;0;0;0;0;0]
      mask Display: e = 0.06;c1 = [120 230 180]/255;c2 = ([120 230 180]+0)/(256+128);c3 = ([120 230 180]+128)/(256+128);patch([0 1 1 0],[0 0 1 1],c1);patch([0 1 1 1-e 1-e 0+e],[0 0 1 1-e 0+e 0+e],c2);patch([0 0 1 1-e 0+e 0+e],[0 1 1 1-e 1-e 0+e],c3);plot([0 1 1 0 0],[0 0 1 1 0]);
  wires:
  "p{1}"/1 -> Delays 1/1("p{1}")
  Delays 1/1("pd{1,1}") -> "IW{1,1}"/1("pd{1,1}")
  "IW{1,1}"/1("iz{1,1}") -> netsum/1
  "b{1}"/1 -> netsum/2
  netsum/1 -> tansig/1
  tansig/1 -> "a{1}"/1

== system DYC_DLCtight_Fuzzy_and_NN_prediction/Function Fitting Neural Network/Layer 2 ==
  "a{1} " : Inport  PortDimensions=20
      mask Display: e = 0.06;c1 = [120 230 180]/255;c2 = ([120 230 180]+0)/(256+128);c3 = ([120 230 180]+128)/(256+128);patch([0 1 1 0],[0 0 1 1],c1);patch([0 1 1 1-e 1-e 0+e],[0 0 1 1-e 0+e 0+e],c2);patch([0 0 1 1-e 0+e 0+e],[0 1 1 1-e 1-e 0+e],c3);plot([0 1 1 0 0],[0 0 1 1 0]);
  Delays 1 : Subsystem
      mask Display: e = 0.06;c1 = [120 150 230]/255;c2 = ([120 150 230]+0)/383;c3 = ([120 150 230]+128)/383;patch([0 1 1 0],[0 0 1 1],c1);patch([0 1 1 1-e 1-e 0+e],[0 0 1 1-e 0+e 0+e],c2);patch([0 0 1 1-e 0+e 0+e],[0 1 1 1-e 1-e 0+e],c3);plot([0 1 1 0 0],[0 0 1 1 0]);disp('0');
  "LW{2,1}" : Subsystem
      mask Display: e = 0.06;c1 = [120 150 230]/255;c2 = ([120 150 230]+0)/383;c3 = ([120 150 230]+128)/383;patch([0 1 1 0],[0 0 1 1],c1);patch([0 1 1 1-e 1-e 0+e],[0 0 1 1-e 0+e 0+e],c2);patch([0 0 1 1-e 0+e 0+e],[0 1 1 1-e 1-e 0+e],c3);plot([0 1 1 0 0],[0 0 1 1 0]);disp('W');
  "b{2}" : Constant  Value=[0.49818218340052339;0.22349560072987809;0.32991448953347441;0.047425267713253241;0.47558601556240288;0.69653904602707184]
      mask Display: e = 0.06;c1 = [120 150 230]/255;c2 = ([120 150 230]+0)/383;c3 = ([120 150 230]+128)/383;patch([0 1 1 0],[0 0 1 1],c1);patch([0 1 1 1-e 1-e 0+e],[0 0 1 1-e 0+e 0+e],c2);patch([0 0 1 1-e 0+e 0+e],[0 1 1 1-e 1-e 0+e],c3);plot([0 1 1 0 0],[0 0 1 1 0]);disp('b');
  netsum : Sum  Inputs=2  SaturateOnIntegerOverflow=on  InputSameDT=on  OutDataTypeStr=Inherit: Same as first input
      mask Display: e = 0.06;c1 = [120 150 230]/255;c2 = ([120 150 230]+0)/383;c3 = ([120 150 230]+128)/383;patch([0 1 1 0],[0 0 1 1],c1);patch([0 1 1 1-e 1-e 0+e],[0 0 1 1-e 0+e 0+e],c2);patch([0 0 1 1-e 0+e 0+e],[0 1 1 1-e 1-e 0+e],c3);plot([0 1 1 0 0],[0 0 1 1 0]);disp('+');
  purelin : neural/Transfer Functions/purelin
  "a{2}" : Outport  InitialOutput=[0;0;0;0;0;0]
      mask Display: e = 0.06;c1 = [120 230 180]/255;c2 = ([120 230 180]+0)/(256+128);c3 = ([120 230 180]+128)/(256+128);patch([0 1 1 0],[0 0 1 1],c1);patch([0 1 1 1-e 1-e 0+e],[0 0 1 1-e 0+e 0+e],c2);patch([0 0 1 1-e 0+e 0+e],[0 1 1 1-e 1-e 0+e],c3);plot([0 1 1 0 0],[0 0 1 1 0]);
  wires:
  "a{1} "/1 -> Delays 1/1("p{2}")
  Delays 1/1("pd{2,1}") -> "LW{2,1}"/1("ad{2,1}")
  "LW{2,1}"/1("lz{2,1}") -> netsum/1
  "b{2}"/1 -> netsum/2
  netsum/1 -> purelin/1
  purelin/1 -> "a{2}"/1

== system DYC_DLCtight_Fuzzy_and_NN_prediction/Function Fitting Neural Network/Process Input 1 ==
  x : Inport  PortDimensions=6
      mask Display: e = 0.06;c1 = [120 230 180]/255;c2 = ([120 230 180]+0)/(256+128);c3 = ([120 230 180]+128)/(256+128);patch([0 1 1 0],[0 0 1 1],c1);patch([0 1 1 1-e 1-e 0+e],[0 0 1 1-e 0+e 0+e],c2);patch([0 0 1 1-e 0+e 0+e],[0 1 1 1-e 1-e 0+e],c3);plot([0 1 1 0 0],[0 0 1 1 0]);
  mapminmax : neural/Processing Functions/mapminmax  xmin=[-5.2337059806962909;-17.716862705801397;-144.17025887640074;30.88118074105488;-4.1986249780184535;-49.245487713955285]  xmax=[4.4066505287036462;18.747488707430712;48.821289964384164;60.000000000000007;3.3670965517122124;37.809970952467388]  ymin=-1  ymax=1
  p : Outport  PortDimensions=6
      mask Display: e = 0.06;c1 = [120 230 180]/255;c2 = ([120 230 180]+0)/(256+128);c3 = ([120 230 180]+128)/(256+128);patch([0 1 1 0],[0 0 1 1],c1);patch([0 1 1 1-e 1-e 0+e],[0 0 1 1-e 0+e 0+e],c2);patch([0 0 1 1-e 0+e 0+e],[0 1 1 1-e 1-e 0+e],c3);plot([0 1 1 0 0],[0 0 1 1 0]);
  wires:
  x/1 -> mapminmax/1
  mapminmax/1 -> p/1

== system DYC_DLCtight_Fuzzy_and_NN_prediction/Function Fitting Neural Network/Process Output 1 ==
  a : Inport  PortDimensions=6
      mask Display: e = 0.06;c1 = [120 230 180]/255;c2 = ([120 230 180]+0)/(256+128);c3 = ([120 230 180]+128)/(256+128);patch([0 1 1 0],[0 0 1 1],c1);patch([0 1 1 1-e 1-e 0+e],[0 0 1 1-e 0+e 0+e],c2);patch([0 0 1 1-e 0+e 0+e],[0 1 1 1-e 1-e 0+e],c3);plot([0 1 1 0 0],[0 0 1 1 0]);
  mapminmax_reverse : neural/Processing Functions/mapminmax_reverse  xmin=[-5.2337059806962909;-17.716862705801397;-144.17025887640074;30.88118074105488;-4.1986249780184535;-49.245487713955285]  xmax=[4.4066505287036462;18.747488707430712;48.821289964384164;60.000000000000007;3.3670965517122124;37.809970952467388]  ymin=-1  ymax=1
  y : Outport  PortDimensions=6
      mask Display: e = 0.06;c1 = [120 230 180]/255;c2 = ([120 230 180]+0)/(256+128);c3 = ([120 230 180]+128)/(256+128);patch([0 1 1 0],[0 0 1 1],c1);patch([0 1 1 1-e 1-e 0+e],[0 0 1 1-e 0+e 0+e],c2);patch([0 0 1 1-e 0+e 0+e],[0 1 1 1-e 1-e 0+e],c3);plot([0 1 1 0 0],[0 0 1 1 0]);
  wires:
  a/1 -> mapminmax_reverse/1
  mapminmax_reverse/1 -> y/1

== system DYC_DLCtight_Fuzzy_and_NN_prediction/Function Fitting Neural Network1/Layer 1 ==
  "p{1}" : Inport  PortDimensions=6
      mask Display: e = 0.06;c1 = [120 230 180]/255;c2 = ([120 230 180]+0)/(256+128);c3 = ([120 230 180]+128)/(256+128);patch([0 1 1 0],[0 0 1 1],c1);patch([0 1 1 1-e 1-e 0+e],[0 0 1 1-e 0+e 0+e],c2);patch([0 0 1 1-e 0+e 0+e],[0 1 1 1-e 1-e 0+e],c3);plot([0 1 1 0 0],[0 0 1 1 0]);
  Delays 1 : Subsystem
      mask Display: e = 0.06;c1 = [120 150 230]/255;c2 = ([120 150 230]+0)/383;c3 = ([120 150 230]+128)/383;patch([0 1 1 0],[0 0 1 1],c1);patch([0 1 1 1-e 1-e 0+e],[0 0 1 1-e 0+e 0+e],c2);patch([0 0 1 1-e 0+e 0+e],[0 1 1 1-e 1-e 0+e],c3);plot([0 1 1 0 0],[0 0 1 1 0]);disp('0');
  "IW{1,1}" : Subsystem
      mask Display: e = 0.06;c1 = [120 150 230]/255;c2 = ([120 150 230]+0)/383;c3 = ([120 150 230]+128)/383;patch([0 1 1 0],[0 0 1 1],c1);patch([0 1 1 1-e 1-e 0+e],[0 0 1 1-e 0+e 0+e],c2);patch([0 0 1 1-e 0+e 0+e],[0 1 1 1-e 1-e 0+e],c3);plot([0 1 1 0 0],[0 0 1 1 0]);disp('W');
  "b{1}" : Constant  Value=[2.6012670118623697;2.1486928926225626;-1.6684480513341911;0.6020839009891702;0.81555962219964073;0.19274185769998825;0.67603470991309556;0.10618126694015399;-0.28052011662375909;-0.7302028865713297;0.98207339265342319;0.75406804357797663;-1.6683908403290786]
      mask Display: e = 0.06;c1 = [120 150 230]/255;c2 = ([120 150 230]+0)/383;c3 = ([120 150 230]+128)/383;patch([0 1 1 0],[0 0 1 1],c1);patch([0 1 1 1-e 1-e 0+e],[0 0 1 1-e 0+e 0+e],c2);patch([0 0 1 1-e 0+e 0+e],[0 1 1 1-e 1-e 0+e],c3);plot([0 1 1 0 0],[0 0 1 1 0]);disp('b');
  netsum : Sum  Inputs=2  SaturateOnIntegerOverflow=on  InputSameDT=on  OutDataTypeStr=Inherit: Same as first input
      mask Display: e = 0.06;c1 = [120 150 230]/255;c2 = ([120 150 230]+0)/383;c3 = ([120 150 230]+128)/383;patch([0 1 1 0],[0 0 1 1],c1);patch([0 1 1 1-e 1-e 0+e],[0 0 1 1-e 0+e 0+e],c2);patch([0 0 1 1-e 0+e 0+e],[0 1 1 1-e 1-e 0+e],c3);plot([0 1 1 0 0],[0 0 1 1 0]);disp('+');
  tansig : neural/Transfer Functions/tansig
  "a{1}" : Outport  InitialOutput=[0;0;0;0;0;0;0;0;0;0;0;0;0]
      mask Display: e = 0.06;c1 = [120 230 180]/255;c2 = ([120 230 180]+0)/(256+128);c3 = ([120 230 180]+128)/(256+128);patch([0 1 1 0],[0 0 1 1],c1);patch([0 1 1 1-e 1-e 0+e],[0 0 1 1-e 0+e 0+e],c2);patch([0 0 1 1-e 0+e 0+e],[0 1 1 1-e 1-e 0+e],c3);plot([0 1 1 0 0],[0 0 1 1 0]);
  wires:
  "p{1}"/1 -> Delays 1/1("p{1}")
  Delays 1/1("pd{1,1}") -> "IW{1,1}"/1("pd{1,1}")
  "IW{1,1}"/1("iz{1,1}") -> netsum/1
  "b{1}"/1 -> netsum/2
  netsum/1 -> tansig/1
  tansig/1 -> "a{1}"/1

== system DYC_DLCtight_Fuzzy_and_NN_prediction/Function Fitting Neural Network1/Layer 2 ==
  "a{1} " : Inport  PortDimensions=13
      mask Display: e = 0.06;c1 = [120 230 180]/255;c2 = ([120 230 180]+0)/(256+128);c3 = ([120 230 180]+128)/(256+128);patch([0 1 1 0],[0 0 1 1],c1);patch([0 1 1 1-e 1-e 0+e],[0 0 1 1-e 0+e 0+e],c2);patch([0 0 1 1-e 0+e 0+e],[0 1 1 1-e 1-e 0+e],c3);plot([0 1 1 0 0],[0 0 1 1 0]);
  Delays 1 : Subsystem
      mask Display: e = 0.06;c1 = [120 150 230]/255;c2 = ([120 150 230]+0)/383;c3 = ([120 150 230]+128)/383;patch([0 1 1 0],[0 0 1 1],c1);patch([0 1 1 1-e 1-e 0+e],[0 0 1 1-e 0+e 0+e],c2);patch([0 0 1 1-e 0+e 0+e],[0 1 1 1-e 1-e 0+e],c3);plot([0 1 1 0 0],[0 0 1 1 0]);disp('0');
  "LW{2,1}" : Subsystem
      mask Display: e = 0.06;c1 = [120 150 230]/255;c2 = ([120 150 230]+0)/383;c3 = ([120 150 230]+128)/383;patch([0 1 1 0],[0 0 1 1],c1);patch([0 1 1 1-e 1-e 0+e],[0 0 1 1-e 0+e 0+e],c2);patch([0 0 1 1-e 0+e 0+e],[0 1 1 1-e 1-e 0+e],c3);plot([0 1 1 0 0],[0 0 1 1 0]);disp('W');
  "b{2}" : Constant  Value=-0.47015434759439723
      mask Display: e = 0.06;c1 = [120 150 230]/255;c2 = ([120 150 230]+0)/383;c3 = ([120 150 230]+128)/383;patch([0 1 1 0],[0 0 1 1],c1);patch([0 1 1 1-e 1-e 0+e],[0 0 1 1-e 0+e 0+e],c2);patch([0 0 1 1-e 0+e 0+e],[0 1 1 1-e 1-e 0+e],c3);plot([0 1 1 0 0],[0 0 1 1 0]);disp('b');
  netsum : Sum  Inputs=2  SaturateOnIntegerOverflow=on  InputSameDT=on  OutDataTypeStr=Inherit: Same as first input
      mask Display: e = 0.06;c1 = [120 150 230]/255;c2 = ([120 150 230]+0)/383;c3 = ([120 150 230]+128)/383;patch([0 1 1 0],[0 0 1 1],c1);patch([0 1 1 1-e 1-e 0+e],[0 0 1 1-e 0+e 0+e],c2);patch([0 0 1 1-e 0+e 0+e],[0 1 1 1-e 1-e 0+e],c3);plot([0 1 1 0 0],[0 0 1 1 0]);disp('+');
  purelin : neural/Transfer Functions/purelin
  "a{2}" : Outport  InitialOutput=0
      mask Display: e = 0.06;c1 = [120 230 180]/255;c2 = ([120 230 180]+0)/(256+128);c3 = ([120 230 180]+128)/(256+128);patch([0 1 1 0],[0 0 1 1],c1);patch([0 1 1 1-e 1-e 0+e],[0 0 1 1-e 0+e 0+e],c2);patch([0 0 1 1-e 0+e 0+e],[0 1 1 1-e 1-e 0+e],c3);plot([0 1 1 0 0],[0 0 1 1 0]);
  wires:
  "a{1} "/1 -> Delays 1/1("p{2}")
  Delays 1/1("pd{2,1}") -> "LW{2,1}"/1("ad{2,1}")
  "LW{2,1}"/1("lz{2,1}") -> netsum/1
  "b{2}"/1 -> netsum/2
  netsum/1 -> purelin/1
  purelin/1 -> "a{2}"/1

== system DYC_DLCtight_Fuzzy_and_NN_prediction/Function Fitting Neural Network1/Process Input 1 ==
  x : Inport  PortDimensions=6
      mask Display: e = 0.06;c1 = [120 230 180]/255;c2 = ([120 230 180]+0)/(256+128);c3 = ([120 230 180]+128)/(256+128);patch([0 1 1 0],[0 0 1 1],c1);patch([0 1 1 1-e 1-e 0+e],[0 0 1 1-e 0+e 0+e],c2);patch([0 0 1 1-e 0+e 0+e],[0 1 1 1-e 1-e 0+e],c3);plot([0 1 1 0 0],[0 0 1 1 0]);
  mapminmax : neural/Processing Functions/mapminmax  xmin=[-5.2337059806962909;-17.716862705801397;-144.17025887640074;30.88118074105488;-4.1986249780184535;-49.245487713955285]  xmax=[4.4066505287036462;18.747488707430712;48.821289964384164;60.000000000000007;3.3670965517122124;37.809970952467388]  ymin=-1  ymax=1
  p : Outport  PortDimensions=6
      mask Display: e = 0.06;c1 = [120 230 180]/255;c2 = ([120 230 180]+0)/(256+128);c3 = ([120 230 180]+128)/(256+128);patch([0 1 1 0],[0 0 1 1],c1);patch([0 1 1 1-e 1-e 0+e],[0 0 1 1-e 0+e 0+e],c2);patch([0 0 1 1-e 0+e 0+e],[0 1 1 1-e 1-e 0+e],c3);plot([0 1 1 0 0],[0 0 1 1 0]);
  wires:
  x/1 -> mapminmax/1
  mapminmax/1 -> p/1

== system DYC_DLCtight_Fuzzy_and_NN_prediction/Function Fitting Neural Network1/Process Output 1 ==
  a : Inport  PortDimensions=1
      mask Display: e = 0.06;c1 = [120 230 180]/255;c2 = ([120 230 180]+0)/(256+128);c3 = ([120 230 180]+128)/(256+128);patch([0 1 1 0],[0 0 1 1],c1);patch([0 1 1 1-e 1-e 0+e],[0 0 1 1-e 0+e 0+e],c2);patch([0 0 1 1-e 0+e 0+e],[0 1 1 1-e 1-e 0+e],c3);plot([0 1 1 0 0],[0 0 1 1 0]);
  mapminmax_reverse : neural/Processing Functions/mapminmax_reverse  xmin=30.88118074105488  xmax=60.000000000000007  ymin=-1  ymax=1
  y : Outport  PortDimensions=1
      mask Display: e = 0.06;c1 = [120 230 180]/255;c2 = ([120 230 180]+0)/(256+128);c3 = ([120 230 180]+128)/(256+128);patch([0 1 1 0],[0 0 1 1],c1);patch([0 1 1 1-e 1-e 0+e],[0 0 1 1-e 0+e 0+e],c2);patch([0 0 1 1-e 0+e 0+e],[0 1 1 1-e 1-e 0+e],c3);plot([0 1 1 0 0],[0 0 1 1 0]);
  wires:
  a/1 -> mapminmax_reverse/1
  mapminmax_reverse/1 -> y/1

== system DYC_DLCtight_Fuzzy_and_NN_prediction/Increment PID /Increment PID  ==
  In1 : Inport
  Delay : Delay  DelayLength=1  InitialCondition=0
  Delay1 : Delay  InitialCondition=0
  Delay2 : Delay  DelayLength=1  InitialCondition=0
  Kd : Gain  Gain=50
  Kp : Gain  Gain=30
  Sum : Sum  Inputs=-+
  Sum1 : Sum  Inputs=-++
  Sum2 : Sum
  Sum3 : Sum
  gain : Gain  Gain=2
  Out1 : Outport
  wires:
  In1/1 -> Sum1/3, Delay1/1, Sum/2, Delay/1
  Delay/1 -> gain/1, Sum/1
  Sum/1 -> Kp/1
  Delay1/1 -> Sum1/2
  Sum1/1 -> Kd/1
  gain/1 -> Sum1/1
  Kp/1 -> Sum2/1
  Kd/1 -> Sum2/2
  Sum2/1 -> Sum3/1
  Sum3/1 -> Delay2/1, Out1/1
  Delay2/1 -> Sum3/2

== system DYC_DLCtight_Fuzzy_and_NN_prediction/NN predictive optimized Fuzzy Control/6I6O Fitting Neural Network1 ==
  Input : Inport  PortDimensions=6
      mask Display: e = 0.06;c1 = [120 230 180]/255;c2 = ([120 230 180]+0)/(256+128);c3 = ([120 230 180]+128)/(256+128);patch([0 1 1 0],[0 0 1 1],c1);patch([0 1 1 1-e 1-e 0+e],[0 0 1 1-e 0+e 0+e],c2);patch([0 0 1 1-e 0+e 0+e],[0 1 1 1-e 1-e 0+e],c3);plot([0 1 1 0 0],[0 0 1 1 0]);
  Layer 1 : Subsystem
      mask Display: e = 0.06;c1 = [120 150 230]/255;c2 = ([120 150 230]+0)/383;c3 = ([120 150 230]+128)/383;patch([0 1 1 0],[0 0 1 1],c1);patch([0 1 1 1-e 1-e 0+e],[0 0 1 1-e 0+e 0+e],c2);patch([0 0 1 1-e 0+e 0+e],[0 1 1 1-e 1-e 0+e],c3);plot([0 1 1 0 0],[0 0 1 1 0]);
  Layer 2 : Subsystem
      mask Display: e = 0.06;c1 = [120 150 230]/255;c2 = ([120 150 230]+0)/383;c3 = ([120 150 230]+128)/383;patch([0 1 1 0],[0 0 1 1],c1);patch([0 1 1 1-e 1-e 0+e],[0 0 1 1-e 0+e 0+e],c2);patch([0 0 1 1-e 0+e 0+e],[0 1 1 1-e 1-e 0+e],c3);plot([0 1 1 0 0],[0 0 1 1 0]);
  Process Input 1 : Subsystem
      mask Display: e = 0.06;c1 = [120 150 230]/255;c2 = ([120 150 230]+0)/383;c3 = ([120 150 230]+128)/383;patch([0 1 1 0],[0 0 1 1],c1);patch([0 1 1 1-e 1-e 0+e],[0 0 1 1-e 0+e 0+e],c2);patch([0 0 1 1-e 0+e 0+e],[0 1 1 1-e 1-e 0+e],c3);plot([0 1 1 0 0],[0 0 1 1 0]);
  Process Output 1 : Subsystem
      mask Display: e = 0.06;c1 = [120 150 230]/255;c2 = ([120 150 230]+0)/383;c3 = ([120 150 230]+128)/383;patch([0 1 1 0],[0 0 1 1],c1);patch([0 1 1 1-e 1-e 0+e],[0 0 1 1-e 0+e 0+e],c2);patch([0 0 1 1-e 0+e 0+e],[0 1 1 1-e 1-e 0+e],c3);plot([0 1 1 0 0],[0 0 1 1 0]);
  Output : Outport  InitialOutput=[0;0;0;0;0;0]
      mask Display: e = 0.06;c1 = [120 230 180]/255;c2 = ([120 230 180]+0)/(256+128);c3 = ([120 230 180]+128)/(256+128);patch([0 1 1 0],[0 0 1 1],c1);patch([0 1 1 1-e 1-e 0+e],[0 0 1 1-e 0+e 0+e],c2);patch([0 0 1 1-e 0+e 0+e],[0 1 1 1-e 1-e 0+e],c3);plot([0 1 1 0 0],[0 0 1 1 0]);
  wires:
  Input/1 -> Process Input 1/1(x)
  Process Output 1/1(y) -> Output/1
  Process Input 1/1(p) -> Layer 1/1("p{1}")
  Layer 1/1("a{1}") -> [feedback1]
  [feedback1] -> Layer 2/1("a{1} ")
  Layer 2/1("a{2}") -> Process Output 1/1(a)

== system DYC_DLCtight_Fuzzy_and_NN_prediction/NN predictive optimized Fuzzy Control/6I6O Fitting Neural Network2 ==
  Input : Inport  PortDimensions=6
      mask Display: e = 0.06;c1 = [120 230 180]/255;c2 = ([120 230 180]+0)/(256+128);c3 = ([120 230 180]+128)/(256+128);patch([0 1 1 0],[0 0 1 1],c1);patch([0 1 1 1-e 1-e 0+e],[0 0 1 1-e 0+e 0+e],c2);patch([0 0 1 1-e 0+e 0+e],[0 1 1 1-e 1-e 0+e],c3);plot([0 1 1 0 0],[0 0 1 1 0]);
  Layer 1 : Subsystem
      mask Display: e = 0.06;c1 = [120 150 230]/255;c2 = ([120 150 230]+0)/383;c3 = ([120 150 230]+128)/383;patch([0 1 1 0],[0 0 1 1],c1);patch([0 1 1 1-e 1-e 0+e],[0 0 1 1-e 0+e 0+e],c2);patch([0 0 1 1-e 0+e 0+e],[0 1 1 1-e 1-e 0+e],c3);plot([0 1 1 0 0],[0 0 1 1 0]);
  Layer 2 : Subsystem
      mask Display: e = 0.06;c1 = [120 150 230]/255;c2 = ([120 150 230]+0)/383;c3 = ([120 150 230]+128)/383;patch([0 1 1 0],[0 0 1 1],c1);patch([0 1 1 1-e 1-e 0+e],[0 0 1 1-e 0+e 0+e],c2);patch([0 0 1 1-e 0+e 0+e],[0 1 1 1-e 1-e 0+e],c3);plot([0 1 1 0 0],[0 0 1 1 0]);
  Process Input 1 : Subsystem
      mask Display: e = 0.06;c1 = [120 150 230]/255;c2 = ([120 150 230]+0)/383;c3 = ([120 150 230]+128)/383;patch([0 1 1 0],[0 0 1 1],c1);patch([0 1 1 1-e 1-e 0+e],[0 0 1 1-e 0+e 0+e],c2);patch([0 0 1 1-e 0+e 0+e],[0 1 1 1-e 1-e 0+e],c3);plot([0 1 1 0 0],[0 0 1 1 0]);
  Process Output 1 : Subsystem
      mask Display: e = 0.06;c1 = [120 150 230]/255;c2 = ([120 150 230]+0)/383;c3 = ([120 150 230]+128)/383;patch([0 1 1 0],[0 0 1 1],c1);patch([0 1 1 1-e 1-e 0+e],[0 0 1 1-e 0+e 0+e],c2);patch([0 0 1 1-e 0+e 0+e],[0 1 1 1-e 1-e 0+e],c3);plot([0 1 1 0 0],[0 0 1 1 0]);
  Output : Outport  InitialOutput=[0;0;0;0;0;0]
      mask Display: e = 0.06;c1 = [120 230 180]/255;c2 = ([120 230 180]+0)/(256+128);c3 = ([120 230 180]+128)/(256+128);patch([0 1 1 0],[0 0 1 1],c1);patch([0 1 1 1-e 1-e 0+e],[0 0 1 1-e 0+e 0+e],c2);patch([0 0 1 1-e 0+e 0+e],[0 1 1 1-e 1-e 0+e],c3);plot([0 1 1 0 0],[0 0 1 1 0]);
  wires:
  Layer 2/1("a{2}") -> Process Output 1/1(a)
  [feedback1] -> Layer 2/1("a{1} ")
  Layer 1/1("a{1}") -> [feedback1]
  Process Input 1/1(p) -> Layer 1/1("p{1}")
  Process Output 1/1(y) -> Output/1
  Input/1 -> Process Input 1/1(x)

== system DYC_DLCtight_Fuzzy_and_NN_prediction/NN predictive optimized Fuzzy Control/6I6O Fitting Neural Network3 ==
  Input : Inport  PortDimensions=6
      mask Display: e = 0.06;c1 = [120 230 180]/255;c2 = ([120 230 180]+0)/(256+128);c3 = ([120 230 180]+128)/(256+128);patch([0 1 1 0],[0 0 1 1],c1);patch([0 1 1 1-e 1-e 0+e],[0 0 1 1-e 0+e 0+e],c2);patch([0 0 1 1-e 0+e 0+e],[0 1 1 1-e 1-e 0+e],c3);plot([0 1 1 0 0],[0 0 1 1 0]);
  Layer 1 : Subsystem
      mask Display: e = 0.06;c1 = [120 150 230]/255;c2 = ([120 150 230]+0)/383;c3 = ([120 150 230]+128)/383;patch([0 1 1 0],[0 0 1 1],c1);patch([0 1 1 1-e 1-e 0+e],[0 0 1 1-e 0+e 0+e],c2);patch([0 0 1 1-e 0+e 0+e],[0 1 1 1-e 1-e 0+e],c3);plot([0 1 1 0 0],[0 0 1 1 0]);
  Layer 2 : Subsystem
      mask Display: e = 0.06;c1 = [120 150 230]/255;c2 = ([120 150 230]+0)/383;c3 = ([120 150 230]+128)/383;patch([0 1 1 0],[0 0 1 1],c1);patch([0 1 1 1-e 1-e 0+e],[0 0 1 1-e 0+e 0+e],c2);patch([0 0 1 1-e 0+e 0+e],[0 1 1 1-e 1-e 0+e],c3);plot([0 1 1 0 0],[0 0 1 1 0]);
  Process Input 1 : Subsystem
      mask Display: e = 0.06;c1 = [120 150 230]/255;c2 = ([120 150 230]+0)/383;c3 = ([120 150 230]+128)/383;patch([0 1 1 0],[0 0 1 1],c1);patch([0 1 1 1-e 1-e 0+e],[0 0 1 1-e 0+e 0+e],c2);patch([0 0 1 1-e 0+e 0+e],[0 1 1 1-e 1-e 0+e],c3);plot([0 1 1 0 0],[0 0 1 1 0]);
  Process Output 1 : Subsystem
      mask Display: e = 0.06;c1 = [120 150 230]/255;c2 = ([120 150 230]+0)/383;c3 = ([120 150 230]+128)/383;patch([0 1 1 0],[0 0 1 1],c1);patch([0 1 1 1-e 1-e 0+e],[0 0 1 1-e 0+e 0+e],c2);patch([0 0 1 1-e 0+e 0+e],[0 1 1 1-e 1-e 0+e],c3);plot([0 1 1 0 0],[0 0 1 1 0]);
  Output : Outport  InitialOutput=[0;0;0;0;0;0]
      mask Display: e = 0.06;c1 = [120 230 180]/255;c2 = ([120 230 180]+0)/(256+128);c3 = ([120 230 180]+128)/(256+128);patch([0 1 1 0],[0 0 1 1],c1);patch([0 1 1 1-e 1-e 0+e],[0 0 1 1-e 0+e 0+e],c2);patch([0 0 1 1-e 0+e 0+e],[0 1 1 1-e 1-e 0+e],c3);plot([0 1 1 0 0],[0 0 1 1 0]);
  wires:
  Input/1 -> Process Input 1/1(x)
  Process Output 1/1(y) -> Output/1
  Process Input 1/1(p) -> Layer 1/1("p{1}")
  Layer 1/1("a{1}") -> [feedback1]
  [feedback1] -> Layer 2/1("a{1} ")
  Layer 2/1("a{2}") -> Process Output 1/1(a)

== system DYC_DLCtight_Fuzzy_and_NN_prediction/NN predictive optimized Fuzzy Control/Fuzzy control ==
  In1 : Inport
  Fuzzy Logic  Controller : fuzblock/Fuzzy Logic  Controller  fis='FuzzyInferenceSystem.fis'
  Gain3 : Gain  Gain=120
  Signal pre-process : Subsystem
  Out1 : Outport
  wires:
  Gain3/1 -> Out1/1
  Signal pre-process/1(Out1) -> Fuzzy Logic  Controller/1
  In1/1 -> Signal pre-process/1(In1)
  Fuzzy Logic  Controller/1 -> Gain3/1

== system DYC_DLCtight_Fuzzy_and_NN_prediction/NN predictive optimized Fuzzy Control/Fuzzy control1 ==
  In1 : Inport
  Fuzzy Logic  Controller : fuzblock/Fuzzy Logic  Controller  fis='FuzzyInferenceSystem.fis'
  Gain3 : Gain  Gain=120
  Signal pre-process : Subsystem
  Out1 : Outport
  wires:
  Fuzzy Logic  Controller/1 -> Gain3/1
  In1/1 -> Signal pre-process/1(In1)
  Signal pre-process/1(Out1) -> Fuzzy Logic  Controller/1
  Gain3/1 -> Out1/1

== system DYC_DLCtight_Fuzzy_and_NN_prediction/NN predictive optimized Fuzzy Control/Fuzzy control2 ==
  In1 : Inport
  Fuzzy Logic  Controller : fuzblock/Fuzzy Logic  Controller  fis='FuzzyInferenceSystem.fis'
  Gain3 : Gain  Gain=120
  Signal pre-process : Subsystem
  Out1 : Outport
  wires:
  Fuzzy Logic  Controller/1 -> Gain3/1
  In1/1 -> Signal pre-process/1(In1)
  Signal pre-process/1(Out1) -> Fuzzy Logic  Controller/1
  Gain3/1 -> Out1/1

== system DYC_DLCtight_Fuzzy_and_NN_prediction/NN predictive optimized Fuzzy Control/Fuzzy control3 ==
  In1 : Inport
  Fuzzy Logic  Controller : fuzblock/Fuzzy Logic  Controller  fis='FuzzyInferenceSystem.fis'
  Gain3 : Gain  Gain=120
  Signal pre-process : Subsystem
  Out1 : Outport
  wires:
  Gain3/1 -> Out1/1
  Signal pre-process/1(Out1) -> Fuzzy Logic  Controller/1
  In1/1 -> Signal pre-process/1(In1)
  Fuzzy Logic  Controller/1 -> Gain3/1

== system DYC_DLCtight_Fuzzy_and_NN_prediction/NN predictive optimized Fuzzy Control/Fuzzy control4 ==
  In1 : Inport
  Fuzzy Logic  Controller : fuzblock/Fuzzy Logic  Controller  fis='FuzzyInferenceSystem.fis'
  Gain3 : Gain  Gain=120
  Signal pre-process : Subsystem
  Out1 : Outport
  wires:
  Gain3/1 -> Out1/1
  Signal pre-process/1(Out1) -> Fuzzy Logic  Controller/1
  In1/1 -> Signal pre-process/1(In1)
  Fuzzy Logic  Controller/1 -> Gain3/1

== system DYC_DLCtight_Fuzzy_and_NN_prediction/ Fuzzy Control/Fuzzy control/Signal pre-process ==
  In1 : Inport
  Delay1 : Delay  DelayLength=1  InitialCondition=0  SampleTime=0.001
  Gain2 : Gain  Gain=0.2
  Gain4 : Gain  Gain=0.2  OutMin=-3  OutMax=3
  Lowpass Filter : dspfdesign/Lowpass Filter  FilterType=FIR  DesignForMinimumOrder=on  FilterOrder=50  PassbandFrequency=0.000001  StopbandFrequency=0.00001  PassbandRipple=0.1  StopbandAttenuation=80  InheritSampleRate=off  SampleRate=0.001  SimulateUsing=Interpreted execution  roundingMode=Floor  coeffsDataTypeStr=fixdt(1,16)
  Mux5 : Mux  Inputs=2
  Saturation : Saturate  UpperLimit=4  LowerLimit=-4
  Saturation1 : Saturate  UpperLimit=4  LowerLimit=-4
  Sum7 : Sum  Inputs=|+-  OutMin=-3  OutMax=3
  Out1 : Outport
  wires:
  Lowpass Filter/1 -> Sum7/2
  Delay1/1 -> Lowpass Filter/1
  Mux5/1 -> Out1/1
  Gain2/1 -> Saturation1/1
  Sum7/1 -> Gain4/1
  Gain4/1 -> Saturation/1
  Saturation/1 -> Mux5/2
  In1/1 -> Delay1/1, Sum7/1, Gain2/1
  Saturation1/1 -> Mux5/1

== system DYC_DLCtight_Fuzzy_and_NN_prediction/Function Fitting Neural Network/Layer 1/Delays 1 ==
  "p{1}" : Inport  PortDimensions=6
      mask Display: e = 0.06;c1 = [120 230 180]/255;c2 = ([120 230 180]+0)/(256+128);c3 = ([120 230 180]+128)/(256+128);patch([0 1 1 0],[0 0 1 1],c1);patch([0 1 1 1-e 1-e 0+e],[0 0 1 1-e 0+e 0+e],c2);patch([0 0 1 1-e 0+e 0+e],[0 1 1 1-e 1-e 0+e],c3);plot([0 1 1 0 0],[0 0 1 1 0]);
  mux : Mux  Inputs=1
      mask Display: e = 0.06;c1 = [120 150 230]/255;c2 = ([120 150 230]+0)/383;c3 = ([120 150 230]+128)/383;patch([0 1 1 0],[0 0 1 1],c1);patch([0 1 1 1-e 1-e 0+e],[0 0 1 1-e 0+e 0+e],c2);patch([0 0 1 1-e 0+e 0+e],[0 1 1 1-e 1-e 0+e],c3);plot([0 1 1 0 0],[0 0 1 1 0]);disp('Mux')
  "pd{1,1}" : Outport
      mask Display: e = 0.06;c1 = [120 230 180]/255;c2 = ([120 230 180]+0)/(256+128);c3 = ([120 230 180]+128)/(256+128);patch([0 1 1 0],[0 0 1 1],c1);patch([0 1 1 1-e 1-e 0+e],[0 0 1 1-e 0+e 0+e],c2);patch([0 0 1 1-e 0+e 0+e],[0 1 1 1-e 1-e 0+e],c3);plot([0 1 1 0 0],[0 0 1 1 0]);
  wires:
  "p{1}"/1 -> mux/1
  mux/1 -> "pd{1,1}"/1
